simulink model "DemoManipulator"  (R2023a)
settings: Solver=ode23t  StartTime=0.0  StopTime=65  MaxStep=0.01  RelTol=1e-3
undefined symbols (not defined in the file): X, Y, Z
libraries: sm_lib x22, nesl_utility x17
settings Model: Creator=KozlovM  LastModifiedBy=Artem Sannikov

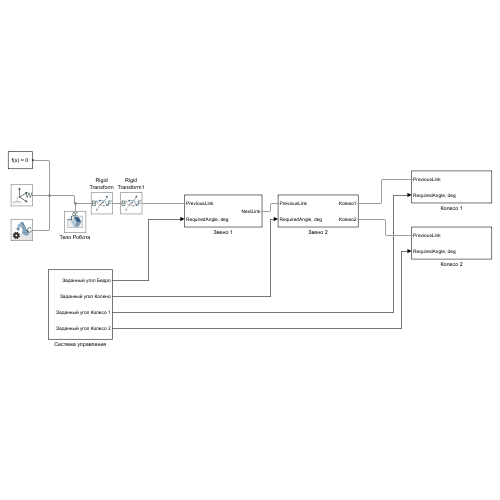
[thumbnail: Simulink's stored preview of the top-level diagram]
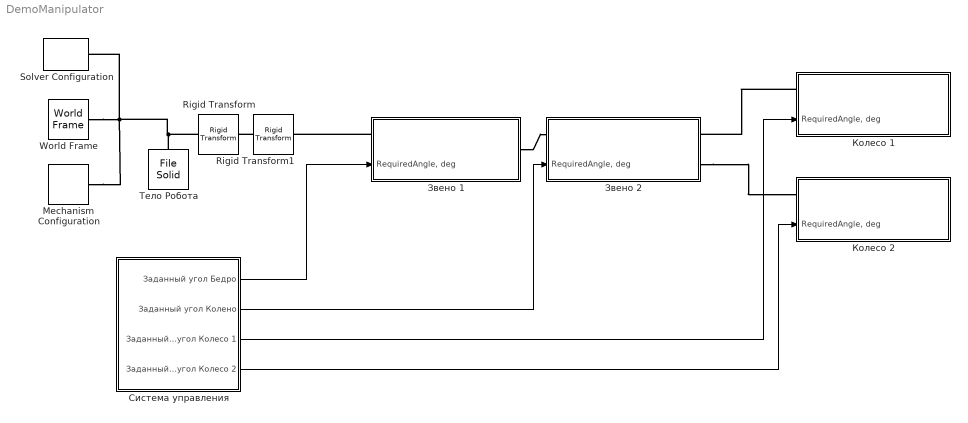
== system DemoManipulator ==
  Mechanism Configuration : sm_lib/Utilities/Mechanism Configuration  UniformGravity=Constant  GravityVector=[0 0 -9.80665]  GravityVectorUnits=m/s^2  LinearizationDelta=0.001  JointModeTransitionNonlinearIterations=2
  Rigid Transform : sm_lib/Frames and Transforms/Rigid Transform  TranslationMethod=StandardAxis  TranslationStandardOffset=117  TranslationStandardOffsetUnits=mm  TranslationStandardAxis=+X  TranslationCartesianOffset=[0 0 0.22]  TranslationCartesianOffsetUnits=m  TranslationROffset=0  TranslationROffsetUnits=m  TranslationZOffset=0  TranslationZOffsetUnits=m  TranslationThetaOffset=0  TranslationThetaOffsetUnits=deg  RotationMethod=None  RotationAngleUnits=deg  RotationStandardAxis=+X  RotationAngle=180  RotationArbitraryAxis=[0 0 1]  FollAlignAxisA=+X  BaseAlignAxisA=+Y  FollAlignAxisB=+Y  BaseAlignAxisB=+Z  RotationSequenceAxes=FollowerAxes  RotationSequence=XYX  RotationSequenceAngles=[0 0 0]  RotationSequenceAnglesUnits=deg  RotationMatrix=[1 0 0; 0 1 0; 0 0 1]  Quaternion=[1 0 0 0]
  Rigid Transform1 : sm_lib/Frames and Transforms/Rigid Transform  TranslationMethod=StandardAxis  TranslationStandardOffset=10  TranslationStandardOffsetUnits=mm  TranslationStandardAxis=-Y  TranslationCartesianOffset=[0 0 0.22]  TranslationCartesianOffsetUnits=m  TranslationROffset=0  TranslationROffsetUnits=m  TranslationZOffset=0  TranslationZOffsetUnits=m  TranslationThetaOffset=0  TranslationThetaOffsetUnits=deg  RotationMethod=None  RotationAngleUnits=deg  RotationStandardAxis=+X  RotationAngle=180  RotationArbitraryAxis=[0 0 1]  FollAlignAxisA=+X  BaseAlignAxisA=+Y  FollAlignAxisB=+Y  BaseAlignAxisB=+Z  RotationSequenceAxes=FollowerAxes  RotationSequence=XYX  RotationSequenceAngles=[0 0 0]  RotationSequenceAnglesUnits=deg  RotationMatrix=[1 0 0; 0 1 0; 0 0 1]  Quaternion=[1 0 0 0]
  Solver Configuration : nesl_utility/Solver Configuration  PhysicalDomain=network_engine_domain  SubClassName=solver  LeftPortType=input  RightPortType=generic  Tones=[]  Harmonics=[]  SimulateNoise=off  Profile=off  UseLocalSampling=off  EnableSwitchedLinearOptims=on  FrequencyDomain=off  UseCCode=off  RelTol=0.001  AbsTol=0.001  MinStep=1e-09  ToWorkspace=off  RevertToSquareIcSolve=off  NumHomotopyIterations=100  PhasorMode=off  PhasorModeNumHarmonics=1  ConsistencySolver=NEWTON_XTOL_AFTER_FTOL  IndexReductionMethod=DerivativeReplacement  DoDC=off  ResidualTolerance=1e-09  ConsistencyTolSource=GLOBAL  ConsistencyAbsTol=0.001  ConsistencyRelTol=0.001  ConsistencyTolFactor=0.001  UseLocalSolver=off  LocalSolverChoice=NE_BACKWARD_EULER_ADVANCER  ResolveIndetEquations=on  FunctionEvalNumThread=1  LocalSolverSampleTime=0.001  DoFixedCost=off  MaxNonlinIter=3  MaxModeIter=2  ComputeImpulses=off  ImpulseIterations=2  LinearAlgebra=auto  LinearAlgebraNumThread=0  EquationFormulation=NE_TIME_EF  DelaysMemoryBudget=1024  AutomaticFiltering=on  FilteringTimeConstant=0.001  PartitionStorageMethod=AS_NEEDED  PartitionMemoryBudget=1024  PartitionMethod=ROBUST
  World Frame : sm_lib/Frames and Transforms/World Frame
  Звено 1 : Subsystem
      settings: PortSchema="{\"entries\":[{\"content\":{\"sides\":[{\"content\":{\"connectorIds\":[\"LConn1\",\"In1\"]},\"type\":\"ConnectorPlacement.EquallySpacedRectSide\",\"uuid\":\"59137c6e-e982-4e9a-8887-9c851b27c4d0\"},{\"content\":{\"connectorIds\":[\"RConn1\"],\"side\":\"RIGHT\"},\"type\":\"ConnectorPlacement.EquallySpacedRectSide\",\"uuid\":\"3006ed02-36e2-47dc-847a-44ef2bf55218\"},{\"content\":{\"side\":\"TOP\"},\"type\":\"ConnectorPlacement.EquallySpacedRectSide\",\"uuid\":\"771aef0a-3ddb-4cfd-8b5b-88211feb2622\"}]},\"type\":\"ConnectorPlacement.EquallySpacedConnector\",\"uuid\":\"e4e6c871-1414-4429-aa1a-adbd621e5483\"}],\"packageUris\":[\"http://schema.mathworks.com/mf0/Connector/R2020b\"],\"version\":\"1.0\"}"
  Звено 2 : Subsystem
      settings: PortSchema="{\"entries\":[{\"content\":{\"sides\":[{\"content\":{\"connectorIds\":[\"LConn1\",\"In1\"]},\"type\":\"ConnectorPlacement.EquallySpacedRectSide\",\"uuid\":\"59137c6e-e982-4e9a-8887-9c851b27c4d0\"},{\"content\":{\"connectorIds\":[\"RConn1\",\"RConn2\"],\"side\":\"RIGHT\"},\"type\":\"ConnectorPlacement.EquallySpacedRectSide\",\"uuid\":\"3006ed02-36e2-47dc-847a-44ef2bf55218\"},{\"content\":{\"side\":\"TOP\"},\"type\":\"ConnectorPlacement.EquallySpacedRectSide\",\"uuid\":\"771aef0a-3ddb-4cfd-8b5b-88211feb2622\"}]},\"type\":\"ConnectorPlacement.EquallySpacedConnector\",\"uuid\":\"e4e6c871-1414-4429-aa1a-adbd621e5483\"}],\"packageUris\":[\"http://schema.mathworks.com/mf0/Connector/R2020b\"],\"version\":\"1.0\"}"
  Колесо 1 : Subsystem
      settings: PortSchema="{\"entries\":[{\"content\":{\"sides\":[{\"content\":{\"connectorIds\":[\"LConn1\",\"In1\"]},\"type\":\"ConnectorPlacement.EquallySpacedRectSide\",\"uuid\":\"59137c6e-e982-4e9a-8887-9c851b27c4d0\"},{\"content\":{\"side\":\"RIGHT\"},\"type\":\"ConnectorPlacement.EquallySpacedRectSide\",\"uuid\":\"3006ed02-36e2-47dc-847a-44ef2bf55218\"},{\"content\":{\"side\":\"TOP\"},\"type\":\"ConnectorPlacement.EquallySpacedRectSide\",\"uuid\":\"771aef0a-3ddb-4cfd-8b5b-88211feb2622\"}]},\"type\":\"ConnectorPlacement.EquallySpacedConnector\",\"uuid\":\"e4e6c871-1414-4429-aa1a-adbd621e5483\"}],\"packageUris\":[\"http://schema.mathworks.com/mf0/Connector/R2020b\"],\"version\":\"1.0\"}"
  Колесо 2 : Subsystem
      settings: PortSchema="{\"entries\":[{\"content\":{\"sides\":[{\"content\":{\"connectorIds\":[\"LConn1\",\"In1\"]},\"type\":\"ConnectorPlacement.EquallySpacedRectSide\",\"uuid\":\"59137c6e-e982-4e9a-8887-9c851b27c4d0\"},{\"content\":{\"side\":\"RIGHT\"},\"type\":\"ConnectorPlacement.EquallySpacedRectSide\",\"uuid\":\"3006ed02-36e2-47dc-847a-44ef2bf55218\"},{\"content\":{\"side\":\"TOP\"},\"type\":\"ConnectorPlacement.EquallySpacedRectSide\",\"uuid\":\"771aef0a-3ddb-4cfd-8b5b-88211feb2622\"}]},\"type\":\"ConnectorPlacement.EquallySpacedConnector\",\"uuid\":\"e4e6c871-1414-4429-aa1a-adbd621e5483\"}],\"packageUris\":[\"http://schema.mathworks.com/mf0/Connector/R2020b\"],\"version\":\"1.0\"}"
  Система управления : Subsystem
  Тело Робота : sm_lib/Body Elements/File Solid  ExtGeomFileName=C:\Users\Artem Sannikov\Desktop\Robo-Forester\Simulink_часть\3D_Models\Body.stp  UnitType=FromFile  ExtGeomFileUnits=ft  StepReaderType=HEX  ExportConvexHullGeometry=off  InertiaType=Custom  Mass=1000  MassUnits=kg  CenterOfMass=[0 0 0]  CenterOfMassUnits=m  MomentsOfInertia=[1 1 1]  MomentsOfInertiaUnits=kg*m^2  ProductsOfInertia=[0 0 0]  ProductsOfInertiaUnits=kg*m^2  BasedOnType=Mass  Density=1000  DensityUnits=kg/m^3  DoExposeReferenceFrame=on  SerializedFrames=<Frames/>  GraphicType=FromGeometry  MarkerShape=Sphere  MarkerSize=10  GraphicVisPropType=SimpleVisualProperties  GraphicDiffuseColor=[0.5 0.5 0.5]  GraphicSpecularColor=[0.5 0.5 0.5 1.0]  GraphicAmbientColor=[0.15 0.15 0.15 1.0]  GraphicEmissiveColor=[0.0 0.0 0.0 1.0]  GraphicShininess=75  GraphicOpacity=1.0
  wires:
  Система управления/1(Заданный угол Бедро) -> Звено 1/1("RequiredAngle, deg")
  Система управления/2(Заданный угол Колено) -> Звено 2/1("RequiredAngle, deg")
  Система управления/3(Заданный угол Колесо 1) -> Колесо 1/1("RequiredAngle, deg")
  Система управления/4(Заданный угол Колесо 2) -> Колесо 2/1("RequiredAngle, deg")
  connections:
  Звено 1/LConn1 -- Rigid Transform1/RConn1
  Звено 1/RConn1 -- Звено 2/LConn1
  Колесо 1/LConn1 -- Звено 2/RConn1
  Rigid Transform/LConn1 -- Mechanism Configuration/RConn1 -- World Frame/RConn1 -- Solver Configuration/RConn1 -- Тело Робота/RConn1
  Rigid Transform1/LConn1 -- Rigid Transform/RConn1
  Звено 2/RConn2 -- Колесо 2/LConn1

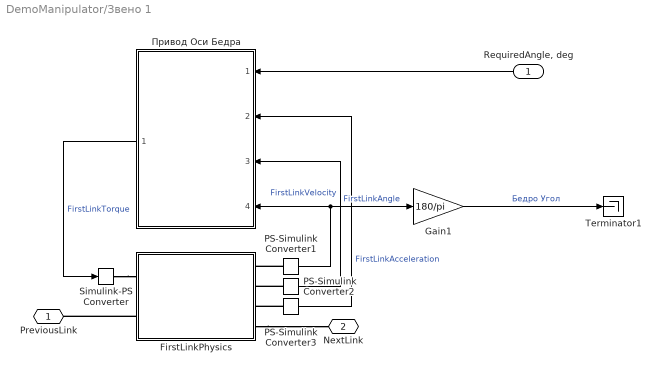
== system DemoManipulator/Звено 1 ==
  "RequiredAngle, deg" : Inport
  FirstLinkPhysics : Subsystem
  Gain1 : Gain  Gain=180/pi
  PS-Simulink Converter1 : nesl_utility/PS-Simulink Converter  PhysicalDomain=network_engine_domain  SubClassName=ps_output  LeftPortType=input  RightPortType=output  PseudoPeriodic=off  Frequencies=[]  VectorFormat=inherit  Unit=inherit  AffineConversion=off
  PS-Simulink Converter2 : nesl_utility/PS-Simulink Converter  PhysicalDomain=network_engine_domain  SubClassName=ps_output  LeftPortType=input  RightPortType=output  PseudoPeriodic=off  Frequencies=[]  VectorFormat=inherit  Unit=inherit  AffineConversion=off
  PS-Simulink Converter3 : nesl_utility/PS-Simulink Converter  PhysicalDomain=network_engine_domain  SubClassName=ps_output  LeftPortType=input  RightPortType=output  PseudoPeriodic=off  Frequencies=[]  VectorFormat=inherit  Unit=inherit  AffineConversion=off
  Simulink-PS Converter : nesl_utility/Simulink-PS Converter  PhysicalDomain=network_engine_domain  SubClassName=ps_input  LeftPortType=input  RightPortType=output  PseudoPeriodic=off  Frequencies=[]  NoiseDistribution=none  NoiseParameters=[]  Unit=1  AffineConversion=off  FilteringAndDerivatives=provide  SimscapeFilterOrder=1  InputFilterTimeConstant=0.001  UdotUserProvided=0
  Terminator1 : Terminator
  Привод Оси Бедра : Subsystem  TreatAsAtomicUnit=on  ReferencedSubsystem=Actuator  K=10  Kv=10  K1=0.05  K2=10  K3=300
  PreviousLink : PMIOPort  Side=Left
  NextLink : PMIOPort  Port=2  Side=Right
  wires:
  Привод Оси Бедра/1 -> Simulink-PS Converter/1  "FirstLinkTorque"
  PS-Simulink Converter1/1 -> Gain1/1, Привод Оси Бедра/4  "FirstLinkAngle"
  PS-Simulink Converter2/1 -> Привод Оси Бедра/3  "FirstLinkVelocity"
  PS-Simulink Converter3/1 -> Привод Оси Бедра/2  "FirstLinkAcceleration"
  "RequiredAngle, deg"/1 -> Привод Оси Бедра/1
  Gain1/1 -> Terminator1/1  "Бедро Угол"
  connections:
  PS-Simulink Converter1/LConn1 -- FirstLinkPhysics/RConn1
  PS-Simulink Converter3/LConn1 -- FirstLinkPhysics/RConn3
  Simulink-PS Converter/RConn1 -- FirstLinkPhysics/LConn1
  PS-Simulink Converter2/LConn1 -- FirstLinkPhysics/RConn2
  FirstLinkPhysics/LConn2 -- PreviousLink/RConn1
  FirstLinkPhysics/RConn4 -- NextLink/RConn1

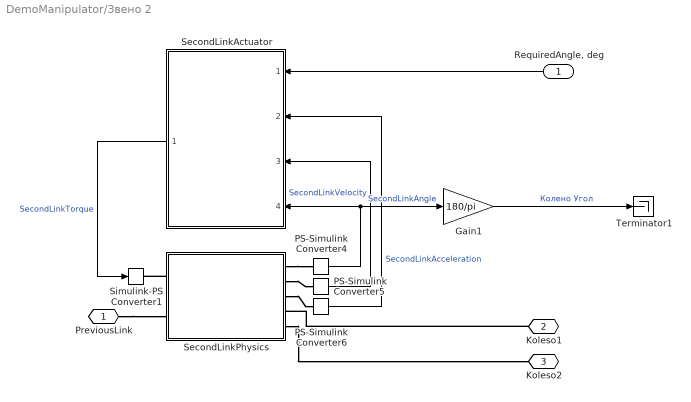
== system DemoManipulator/Звено 2 ==
  "RequiredAngle, deg" : Inport
  Gain1 : Gain  Gain=180/pi
  PS-Simulink Converter4 : nesl_utility/PS-Simulink Converter  PhysicalDomain=network_engine_domain  SubClassName=ps_output  LeftPortType=input  RightPortType=output  PseudoPeriodic=off  Frequencies=[]  VectorFormat=inherit  Unit=inherit  AffineConversion=off
  PS-Simulink Converter5 : nesl_utility/PS-Simulink Converter  PhysicalDomain=network_engine_domain  SubClassName=ps_output  LeftPortType=input  RightPortType=output  PseudoPeriodic=off  Frequencies=[]  VectorFormat=inherit  Unit=inherit  AffineConversion=off
  PS-Simulink Converter6 : nesl_utility/PS-Simulink Converter  PhysicalDomain=network_engine_domain  SubClassName=ps_output  LeftPortType=input  RightPortType=output  PseudoPeriodic=off  Frequencies=[]  VectorFormat=inherit  Unit=inherit  AffineConversion=off
  SecondLinkActuator : Subsystem  TreatAsAtomicUnit=on  ReferencedSubsystem=Actuator  K=10  Kv=15  K1=0.05  K2=50  K3=100
  SecondLinkPhysics : Subsystem
  Simulink-PS Converter1 : nesl_utility/Simulink-PS Converter  PhysicalDomain=network_engine_domain  SubClassName=ps_input  LeftPortType=input  RightPortType=output  PseudoPeriodic=off  Frequencies=[]  NoiseDistribution=none  NoiseParameters=[]  Unit=1  AffineConversion=off  FilteringAndDerivatives=provide  SimscapeFilterOrder=1  InputFilterTimeConstant=0.001  UdotUserProvided=0
  Terminator1 : Terminator
  PreviousLink : PMIOPort  Side=Left
  Koleso1 : PMIOPort  Port=2  Side=Right
  Koleso2 : PMIOPort  Port=3  Side=Right
  wires:
  SecondLinkActuator/1 -> Simulink-PS Converter1/1  "SecondLinkTorque"
  PS-Simulink Converter5/1 -> SecondLinkActuator/3  "SecondLinkVelocity"
  PS-Simulink Converter6/1 -> SecondLinkActuator/2  "SecondLinkAcceleration"
  "RequiredAngle, deg"/1 -> SecondLinkActuator/1
  Gain1/1 -> Terminator1/1  "Колено Угол"
  PS-Simulink Converter4/1 -> SecondLinkActuator/4, Gain1/1  "SecondLinkAngle"
  connections:
  SecondLinkPhysics/RConn1 -- PS-Simulink Converter4/LConn1
  SecondLinkPhysics/RConn2 -- PS-Simulink Converter5/LConn1
  SecondLinkPhysics/LConn1 -- Simulink-PS Converter1/RConn1
  SecondLinkPhysics/RConn3 -- PS-Simulink Converter6/LConn1
  Koleso1/RConn1 -- SecondLinkPhysics/RConn4
  PreviousLink/RConn1 -- SecondLinkPhysics/LConn2
  SecondLinkPhysics/RConn5 -- Koleso2/RConn1

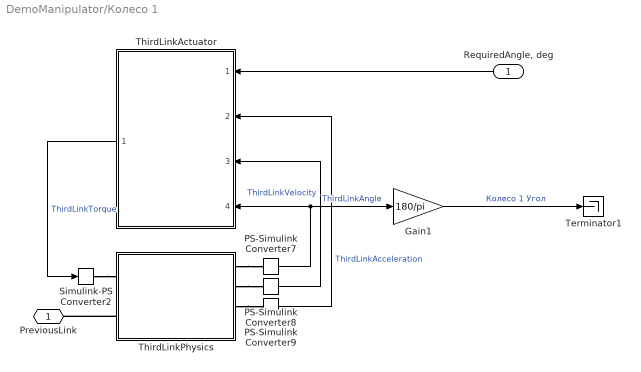
== system DemoManipulator/Колесо 1 ==
  "RequiredAngle, deg" : Inport
  Gain1 : Gain  Gain=180/pi
  PS-Simulink Converter7 : nesl_utility/PS-Simulink Converter  PhysicalDomain=network_engine_domain  SubClassName=ps_output  LeftPortType=input  RightPortType=output  PseudoPeriodic=off  Frequencies=[]  VectorFormat=inherit  Unit=inherit  AffineConversion=off
  PS-Simulink Converter8 : nesl_utility/PS-Simulink Converter  PhysicalDomain=network_engine_domain  SubClassName=ps_output  LeftPortType=input  RightPortType=output  PseudoPeriodic=off  Frequencies=[]  VectorFormat=inherit  Unit=inherit  AffineConversion=off
  PS-Simulink Converter9 : nesl_utility/PS-Simulink Converter  PhysicalDomain=network_engine_domain  SubClassName=ps_output  LeftPortType=input  RightPortType=output  PseudoPeriodic=off  Frequencies=[]  VectorFormat=inherit  Unit=inherit  AffineConversion=off
  Simulink-PS Converter2 : nesl_utility/Simulink-PS Converter  PhysicalDomain=network_engine_domain  SubClassName=ps_input  LeftPortType=input  RightPortType=output  PseudoPeriodic=off  Frequencies=[]  NoiseDistribution=none  NoiseParameters=[]  Unit=1  AffineConversion=off  FilteringAndDerivatives=provide  SimscapeFilterOrder=1  InputFilterTimeConstant=0.001  UdotUserProvided=0
  Terminator1 : Terminator
  ThirdLinkActuator : Subsystem  TreatAsAtomicUnit=on  ReferencedSubsystem=Actuator  K=10  Kv=10  K1=0.05  K2=10  K3=1000
  ThirdLinkPhysics : Subsystem
  PreviousLink : PMIOPort  Side=Left
  wires:
  ThirdLinkActuator/1 -> Simulink-PS Converter2/1  "ThirdLinkTorque"
  PS-Simulink Converter7/1 -> Gain1/1, ThirdLinkActuator/4  "ThirdLinkAngle"
  PS-Simulink Converter9/1 -> ThirdLinkActuator/2  "ThirdLinkAcceleration"
  PS-Simulink Converter8/1 -> ThirdLinkActuator/3  "ThirdLinkVelocity"
  Gain1/1 -> Terminator1/1  "Колесо 1 Угол"
  "RequiredAngle, deg"/1 -> ThirdLinkActuator/1
  connections:
  ThirdLinkPhysics/RConn3 -- PS-Simulink Converter9/LConn1
  Simulink-PS Converter2/RConn1 -- ThirdLinkPhysics/LConn1
  ThirdLinkPhysics/RConn2 -- PS-Simulink Converter8/LConn1
  ThirdLinkPhysics/RConn1 -- PS-Simulink Converter7/LConn1
  ThirdLinkPhysics/LConn2 -- PreviousLink/RConn1

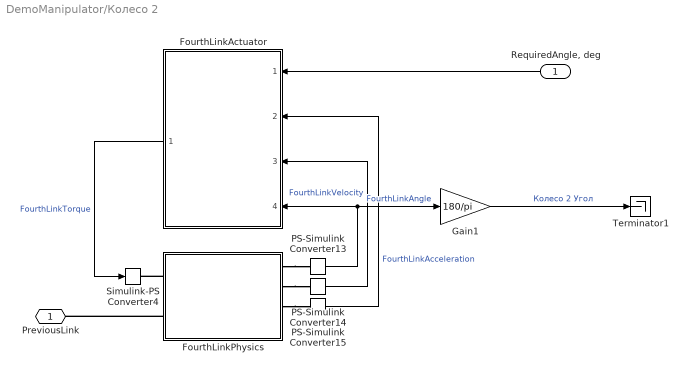
== system DemoManipulator/Колесо 2 ==
  "RequiredAngle, deg" : Inport
  FourthLinkActuator : Subsystem  TreatAsAtomicUnit=on  ReferencedSubsystem=Actuator  K=10  Kv=10  K1=0.05  K2=10  K3=100
  FourthLinkPhysics : Subsystem
  Gain1 : Gain  Gain=180/pi
  PS-Simulink Converter13 : nesl_utility/PS-Simulink Converter  PhysicalDomain=network_engine_domain  SubClassName=ps_output  LeftPortType=input  RightPortType=output  PseudoPeriodic=off  Frequencies=[]  VectorFormat=inherit  Unit=inherit  AffineConversion=off
  PS-Simulink Converter14 : nesl_utility/PS-Simulink Converter  PhysicalDomain=network_engine_domain  SubClassName=ps_output  LeftPortType=input  RightPortType=output  PseudoPeriodic=off  Frequencies=[]  VectorFormat=inherit  Unit=inherit  AffineConversion=off
  PS-Simulink Converter15 : nesl_utility/PS-Simulink Converter  PhysicalDomain=network_engine_domain  SubClassName=ps_output  LeftPortType=input  RightPortType=output  PseudoPeriodic=off  Frequencies=[]  VectorFormat=inherit  Unit=inherit  AffineConversion=off
  Simulink-PS Converter4 : nesl_utility/Simulink-PS Converter  PhysicalDomain=network_engine_domain  SubClassName=ps_input  LeftPortType=input  RightPortType=output  PseudoPeriodic=off  Frequencies=[]  NoiseDistribution=none  NoiseParameters=[]  Unit=1  AffineConversion=off  FilteringAndDerivatives=provide  SimscapeFilterOrder=1  InputFilterTimeConstant=0.001  UdotUserProvided=0
  Terminator1 : Terminator
  PreviousLink : PMIOPort  Side=Left
  wires:
  FourthLinkActuator/1 -> Simulink-PS Converter4/1  "FourthLinkTorque"
  PS-Simulink Converter14/1 -> FourthLinkActuator/3  "FourthLinkVelocity"
  PS-Simulink Converter15/1 -> FourthLinkActuator/2  "FourthLinkAcceleration"
  Gain1/1 -> Terminator1/1  "Колесо 2 Угол"
  PS-Simulink Converter13/1 -> FourthLinkActuator/4, Gain1/1  "FourthLinkAngle"
  "RequiredAngle, deg"/1 -> FourthLinkActuator/1
  connections:
  FourthLinkPhysics/LConn1 -- Simulink-PS Converter4/RConn1
  FourthLinkPhysics/RConn2 -- PS-Simulink Converter14/LConn1
  FourthLinkPhysics/RConn1 -- PS-Simulink Converter13/LConn1
  FourthLinkPhysics/RConn3 -- PS-Simulink Converter15/LConn1
  FourthLinkPhysics/LConn2 -- PreviousLink/RConn1

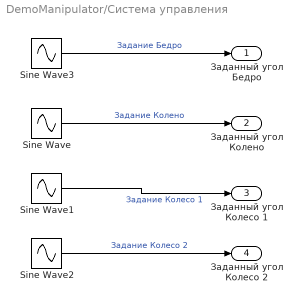
== system DemoManipulator/Система управления ==
  Sine Wave : Sin  Amplitude=180  Bias=60  Frequency=0.5  SampleTime=0
  Sine Wave1 : Sin  Amplitude=30  Bias=40  SampleTime=0
  Sine Wave2 : Sin  Amplitude=30  Bias=40  SampleTime=0
  Sine Wave3 : Sin  Amplitude=40  Bias=60  Frequency=0.5  SampleTime=0
  Заданный угол Бедро : Outport
  Заданный угол Колено : Outport  Port=2
  Заданный угол Колесо 1 : Outport  Port=3
  Заданный угол Колесо 2 : Outport  Port=4
  wires:
  Sine Wave/1 -> Заданный угол Колено/1  "Задание Колено"
  Sine Wave3/1 -> Заданный угол Бедро/1  "Задание Бедро"
  Sine Wave2/1 -> Заданный угол Колесо 2/1  "Задание Колесо 2"
  Sine Wave1/1 -> Заданный угол Колесо 1/1  "Задание Колесо 1"

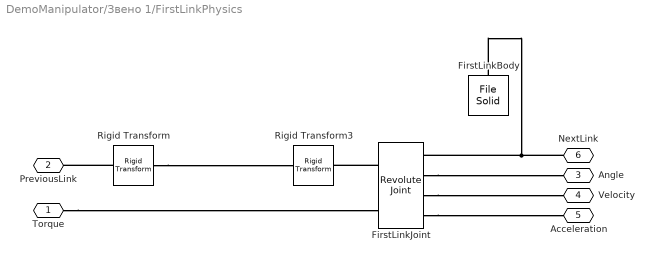
== system DemoManipulator/Звено 1/FirstLinkPhysics ==
  FirstLinkBody : sm_lib/Body Elements/File Solid  ExtGeomFileName=C:\Users\Artem Sannikov\Desktop\Robo-Forester\Simulink_часть\3D_Models\Leg.stp  UnitType=FromFile  ExtGeomFileUnits=m  StepReaderType=HEX  ExportConvexHullGeometry=off  InertiaType=Custom  Mass=5.3  MassUnits=kg  CenterOfMass=[0 0 -90]  CenterOfMassUnits=mm  MomentsOfInertia=[15.3 20.5 5.7]  MomentsOfInertiaUnits=kg*m^2  ProductsOfInertia=[0 0 0]  ProductsOfInertiaUnits=kg*m^2  BasedOnType=DensityFromFile  Density=1000  DensityUnits=kg/m^3  DoExposeReferenceFrame=on  SerializedFrames=<Frames><Frame><Id>Frame1</Id><Value><Name>Bedro</Name><Origin><Source>GeometricFeature</Source><FeatureName>cylindrical surface 7</FeatureName></Origin><PrimaryAxis><DefinedDirection>+Z</DefinedDirection><Source>GeometricFeature</Source><SourceDirection>+Z</SourceDirection><FeatureName>cylindrical surface 7</FeatureName></PrimaryAxis><SecondaryAxis><DefinedDirection>+X</DefinedDirection><Source>GeometricFeature</Source><SourceDirection>+X</SourceDirection><FeatureName></FeatureName></SecondaryAxis></Value></Frame></Frames>  GraphicType=FromGeometry  MarkerShape=Sphere  MarkerSize=10  GraphicVisPropType=FromFileVisualProperties  GraphicDiffuseColor=[0.5 0.5 0.5]  GraphicSpecularColor=[0.5 0.5 0.5 1.0]  GraphicAmbientColor=[0.15 0.15 0.15 1.0]  GraphicEmissiveColor=[0.0 0.0 0.0 1.0]  GraphicShininess=75  GraphicOpacity=1.0
  FirstLinkJoint : sm_lib/Joints/Revolute Joint  JointMode=Normal  SenseConstraintForce=off  SenseConstraintForceX=off  SenseConstraintForceY=off  SenseConstraintForceZ=off  SenseConstraintTorque=off  SenseConstraintTorqueX=off  SenseConstraintTorqueY=off  SenseConstraintTorqueZ=off  SenseTotalForce=off  SenseTotalForceX=off  SenseTotalForceY=off  SenseTotalForceZ=off  SenseTotalTorque=off  SenseTotalTorqueX=off  SenseTotalTorqueY=off  SenseTotalTorqueZ=off  CompositeWrenchDir=FollowerOnBase  CompositeWrenchFrame=BaseFrame  EquilibriumPosition=0  EquilibriumPositionUnits=deg  SpringStiffness=0  SpringStiffnessUnits=N*m/deg  DampingCoefficient=0.1  DampingCoefficientUnits=N*m/(deg/s)  TorqueActuationMode=InputTorque  MotionActuationMode=ComputedMotion  SensePosition=on  SenseVelocity=on  SenseAcceleration=on  SenseTorqueForce=off  SenseLowerLimitTorqueForce=off  SenseUpperLimitTorqueForce=off  LowerLimitSpecify=on  LowerLimitBound=-170  LowerLimitBoundUnits=deg  LowerLimitStiffness=1e4  LowerLimitStiffnessUnits=N*m/deg  LowerLimitDamping=1000  LowerLimitDampingUnits=N*m/(deg/s)  LowerLimitTransitionRegionWidth=0.1  LowerLimitTransitionRegionWidthUnits=deg  UpperLimitSpecify=on  UpperLimitBound=170  UpperLimitBoundUnits=deg  UpperLimitStiffness=1e4  UpperLimitStiffnessUnits=N*m/deg  UpperLimitDamping=1000  UpperLimitDampingUnits=N*m/(deg/s)  UpperLimitTransitionRegionWidth=0.1  UpperLimitTransitionRegionWidthUnits=deg  PositionTargetSpecify=on  PositionTargetPriority=High  PositionTargetValue=0  PositionTargetValueUnits=deg  VelocityTargetSpecify=off  VelocityTargetPriority=High  VelocityTargetValue=0  VelocityTargetValueUnits=deg/s
  Rigid Transform : sm_lib/Frames and Transforms/Rigid Transform  TranslationMethod=None  TranslationStandardOffset=0  TranslationStandardOffsetUnits=m  TranslationStandardAxis=+Z  TranslationCartesianOffset=[0 0 0.22]  TranslationCartesianOffsetUnits=m  TranslationROffset=0  TranslationROffsetUnits=m  TranslationZOffset=0  TranslationZOffsetUnits=m  TranslationThetaOffset=0  TranslationThetaOffsetUnits=deg  RotationMethod=StandardAxis  RotationAngleUnits=deg  RotationStandardAxis=-Z  RotationAngle=45  RotationArbitraryAxis=[0 0 1]  FollAlignAxisA=+X  BaseAlignAxisA=+Y  FollAlignAxisB=+Y  BaseAlignAxisB=+Z  RotationSequenceAxes=FollowerAxes  RotationSequence=XYX  RotationSequenceAngles=[0 0 0]  RotationSequenceAnglesUnits=deg  RotationMatrix=[1 0 0; 0 1 0; 0 0 1]  Quaternion=[1 0 0 0]
  Rigid Transform3 : sm_lib/Frames and Transforms/Rigid Transform  TranslationMethod=StandardAxis  TranslationStandardOffset=10  TranslationStandardOffsetUnits=mm  TranslationStandardAxis=+Z  TranslationCartesianOffset=[0 0 0.22]  TranslationCartesianOffsetUnits=m  TranslationROffset=0  TranslationROffsetUnits=m  TranslationZOffset=0  TranslationZOffsetUnits=m  TranslationThetaOffset=0  TranslationThetaOffsetUnits=deg  RotationMethod=None  RotationAngleUnits=deg  RotationStandardAxis=+X  RotationAngle=180  RotationArbitraryAxis=[0 0 1]  FollAlignAxisA=+X  BaseAlignAxisA=+Y  FollAlignAxisB=+Y  BaseAlignAxisB=+Z  RotationSequenceAxes=FollowerAxes  RotationSequence=XYX  RotationSequenceAngles=[0 0 0]  RotationSequenceAnglesUnits=deg  RotationMatrix=[1 0 0; 0 1 0; 0 0 1]  Quaternion=[1 0 0 0]
  Torque : PMIOPort  Side=Left
  PreviousLink : PMIOPort  Port=2  Side=Left
  Angle : PMIOPort  Port=3  Side=Right
  Velocity : PMIOPort  Port=4  Side=Right
  Acceleration : PMIOPort  Port=5  Side=Right
  NextLink : PMIOPort  Port=6  Side=Right
  connections:
  FirstLinkJoint/RConn2 -- Angle/RConn1
  FirstLinkJoint/RConn4 -- Acceleration/RConn1
  FirstLinkJoint/RConn3 -- Velocity/RConn1
  NextLink/RConn1 -- FirstLinkBody/LConn1 -- FirstLinkJoint/RConn1
  FirstLinkJoint/LConn1 -- Rigid Transform3/RConn1
  Torque/RConn1 -- FirstLinkJoint/LConn2
  Rigid Transform/LConn1 -- PreviousLink/RConn1
  Rigid Transform/RConn1 -- Rigid Transform3/LConn1

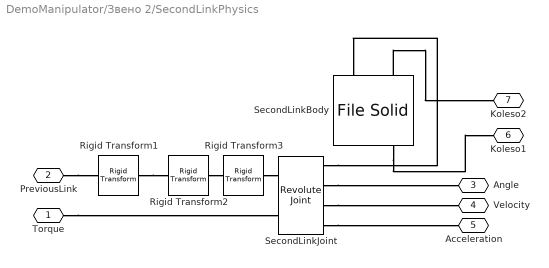
== system DemoManipulator/Звено 2/SecondLinkPhysics ==
  Rigid Transform1 : sm_lib/Frames and Transforms/Rigid Transform  TranslationMethod=StandardAxis  TranslationStandardOffset=110  TranslationStandardOffsetUnits=mm  TranslationStandardAxis=-Y  TranslationCartesianOffset=[0 0 0.22]  TranslationCartesianOffsetUnits=m  TranslationROffset=0  TranslationROffsetUnits=m  TranslationZOffset=0  TranslationZOffsetUnits=m  TranslationThetaOffset=0  TranslationThetaOffsetUnits=deg  RotationMethod=None  RotationAngleUnits=deg  RotationStandardAxis=+X  RotationAngle=180  RotationArbitraryAxis=[0 0 1]  FollAlignAxisA=+X  BaseAlignAxisA=+Y  FollAlignAxisB=+Y  BaseAlignAxisB=+Z  RotationSequenceAxes=FollowerAxes  RotationSequence=XYX  RotationSequenceAngles=[0 0 0]  RotationSequenceAnglesUnits=deg  RotationMatrix=[1 0 0; 0 1 0; 0 0 1]  Quaternion=[1 0 0 0]
  Rigid Transform2 : sm_lib/Frames and Transforms/Rigid Transform  TranslationMethod=StandardAxis  TranslationStandardOffset=221  TranslationStandardOffsetUnits=mm  TranslationStandardAxis=-X  TranslationCartesianOffset=[0 0 0.22]  TranslationCartesianOffsetUnits=m  TranslationROffset=0  TranslationROffsetUnits=m  TranslationZOffset=0  TranslationZOffsetUnits=m  TranslationThetaOffset=0  TranslationThetaOffsetUnits=deg  RotationMethod=None  RotationAngleUnits=deg  RotationStandardAxis=+X  RotationAngle=180  RotationArbitraryAxis=[0 0 1]  FollAlignAxisA=+X  BaseAlignAxisA=+Y  FollAlignAxisB=+Y  BaseAlignAxisB=+Z  RotationSequenceAxes=FollowerAxes  RotationSequence=XYX  RotationSequenceAngles=[0 0 0]  RotationSequenceAnglesUnits=deg  RotationMatrix=[1 0 0; 0 1 0; 0 0 1]  Quaternion=[1 0 0 0]
  Rigid Transform3 : sm_lib/Frames and Transforms/Rigid Transform  TranslationMethod=StandardAxis  TranslationStandardOffset=75  TranslationStandardOffsetUnits=mm  TranslationStandardAxis=-Z  TranslationCartesianOffset=[0 0 0.22]  TranslationCartesianOffsetUnits=m  TranslationROffset=0  TranslationROffsetUnits=m  TranslationZOffset=0  TranslationZOffsetUnits=m  TranslationThetaOffset=0  TranslationThetaOffsetUnits=deg  RotationMethod=None  RotationAngleUnits=deg  RotationStandardAxis=+X  RotationAngle=180  RotationArbitraryAxis=[0 0 1]  FollAlignAxisA=+X  BaseAlignAxisA=+Y  FollAlignAxisB=+Y  BaseAlignAxisB=+Z  RotationSequenceAxes=FollowerAxes  RotationSequence=XYX  RotationSequenceAngles=[0 0 0]  RotationSequenceAnglesUnits=deg  RotationMatrix=[1 0 0; 0 1 0; 0 0 1]  Quaternion=[1 0 0 0]
  SecondLinkBody : sm_lib/Body Elements/File Solid  ExtGeomFileName=C:\Users\Artem Sannikov\Desktop\Robo-Forester\Simulink_часть\3D_Models\knee.stp  UnitType=FromFile  ExtGeomFileUnits=m  StepReaderType=HEX  ExportConvexHullGeometry=off  InertiaType=Custom  Mass=2  MassUnits=kg  CenterOfMass=[-100 0 0]  CenterOfMassUnits=mm  MomentsOfInertia=[13.4 18.7 6.4]  MomentsOfInertiaUnits=kg*m^2  ProductsOfInertia=[0 0 0]  ProductsOfInertiaUnits=kg*m^2  BasedOnType=DensityFromFile  Density=1000  DensityUnits=kg/m^3  DoExposeReferenceFrame=on  SerializedFrames=<Frames><Frame><Id>Frame1</Id><Value><Name>Koleno</Name><Origin><Source>GeometricFeature</Source><FeatureName>planar surface 1</FeatureName></Origin><PrimaryAxis><DefinedDirection>+Z</DefinedDirection><Source>GeometricFeature</Source><SourceDirection>+Z</SourceDirection><FeatureName>planar surface 1</FeatureName></PrimaryAxis><SecondaryAxis><DefinedDirection>+X</DefinedDirection><Source>ReferenceFrame</Source><SourceDirection>+X</SourceDirection><FeatureName></FeatureName></SecondaryAxis></Value></Frame><Frame><Id>Frame2</Id><Value><Name>Koleso2</Name><Origin><Source>GeometricFeature</Source><FeatureName>planar surface 2</FeatureName></Origin><PrimaryAxis><DefinedDirection>+Z</DefinedDirection><Source>ReferenceFrame</Source><SourceDirection>+Z</SourceDirection><FeatureName></FeatureName></PrimaryAxis><SecondaryAxis><DefinedDirection>+X</DefinedDirection><Source>ReferenceFrame</Source><SourceDirection>+X</SourceDirection><FeatureName></FeatureName></SecondaryAxis></Value></Frame><Frame><Id>Frame3</Id><Value><Name>Koleso1</Name><Origin><Source>GeometricFeature</Source><FeatureName>planar surface 7</FeatureName></Origin><PrimaryAxis><DefinedDirection>+Z</DefinedDirection><Source>ReferenceFrame</Source><SourceDirection>+Z</SourceDirection><FeatureName></FeatureName></PrimaryAxis><SecondaryAxis><DefinedDirection>+X</DefinedDirection><Source>ReferenceFrame</Source><SourceDirection>+X</SourceDirection><FeatureName></FeatureName></SecondaryAxis></Value></Frame></Frames>  GraphicType=FromGeometry  MarkerShape=Sphere  MarkerSize=10  GraphicVisPropType=SimpleVisualProperties  GraphicDiffuseColor=[0.5 0.5 0.5]  GraphicSpecularColor=[0.5 0.5 0.5 1.0]  GraphicAmbientColor=[0.15 0.15 0.15 1.0]  GraphicEmissiveColor=[0.0 0.0 0.0 1.0]  GraphicShininess=75  GraphicOpacity=1.0
  SecondLinkJoint : sm_lib/Joints/Revolute Joint  JointMode=Normal  SenseConstraintForce=off  SenseConstraintForceX=off  SenseConstraintForceY=off  SenseConstraintForceZ=off  SenseConstraintTorque=off  SenseConstraintTorqueX=off  SenseConstraintTorqueY=off  SenseConstraintTorqueZ=off  SenseTotalForce=off  SenseTotalForceX=off  SenseTotalForceY=off  SenseTotalForceZ=off  SenseTotalTorque=off  SenseTotalTorqueX=off  SenseTotalTorqueY=off  SenseTotalTorqueZ=off  CompositeWrenchDir=FollowerOnBase  CompositeWrenchFrame=BaseFrame  EquilibriumPosition=0  EquilibriumPositionUnits=deg  SpringStiffness=0  SpringStiffnessUnits=N*m/deg  DampingCoefficient=0.1  DampingCoefficientUnits=N*m/(deg/s)  TorqueActuationMode=InputTorque  MotionActuationMode=ComputedMotion  SensePosition=on  SenseVelocity=on  SenseAcceleration=on  SenseTorqueForce=off  SenseLowerLimitTorqueForce=off  SenseUpperLimitTorqueForce=off  LowerLimitSpecify=on  LowerLimitBound=-170  LowerLimitBoundUnits=deg  LowerLimitStiffness=1e4  LowerLimitStiffnessUnits=N*m/deg  LowerLimitDamping=1000  LowerLimitDampingUnits=N*m/(deg/s)  LowerLimitTransitionRegionWidth=0.1  LowerLimitTransitionRegionWidthUnits=deg  UpperLimitSpecify=on  UpperLimitBound=50  UpperLimitBoundUnits=deg  UpperLimitStiffness=1e4  UpperLimitStiffnessUnits=N*m/deg  UpperLimitDamping=10  UpperLimitDampingUnits=N*m/(deg/s)  UpperLimitTransitionRegionWidth=0.1  UpperLimitTransitionRegionWidthUnits=deg  PositionTargetSpecify=on  PositionTargetPriority=High  PositionTargetValue=-90  PositionTargetValueUnits=deg  VelocityTargetSpecify=off  VelocityTargetPriority=High  VelocityTargetValue=0  VelocityTargetValueUnits=deg/s
  Torque : PMIOPort  Side=Left
  PreviousLink : PMIOPort  Port=2  Side=Left
  Angle : PMIOPort  Port=3  Side=Right
  Velocity : PMIOPort  Port=4  Side=Right
  Acceleration : PMIOPort  Port=5  Side=Right
  Koleso1 : PMIOPort  Port=6  Side=Right
  Koleso2 : PMIOPort  Port=7  Side=Right
  connections:
  SecondLinkJoint/RConn2 -- Angle/RConn1
  SecondLinkJoint/RConn4 -- Acceleration/RConn1
  SecondLinkJoint/RConn3 -- Velocity/RConn1
  SecondLinkJoint/RConn1 -- SecondLinkBody/LConn1
  Rigid Transform2/RConn1 -- Rigid Transform3/LConn1
  Torque/RConn1 -- SecondLinkJoint/LConn2
  PreviousLink/RConn1 -- Rigid Transform1/LConn1
  Rigid Transform1/RConn1 -- Rigid Transform2/LConn1
  Rigid Transform3/RConn1 -- SecondLinkJoint/LConn1
  SecondLinkBody/LConn2 -- Koleso2/RConn1
  SecondLinkBody/RConn2 -- Koleso1/RConn1

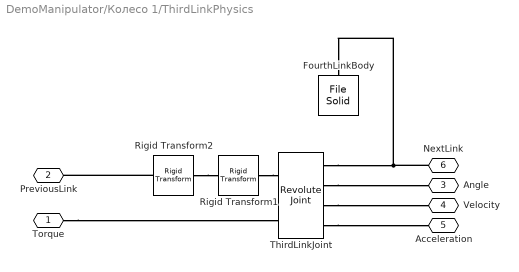
== system DemoManipulator/Колесо 1/ThirdLinkPhysics ==
  FourthLinkBody : sm_lib/Body Elements/File Solid  ExtGeomFileName=C:\Users\Artem Sannikov\Desktop\Robo-Forester\Simulink_часть\3D_Models\Wheel.stp  UnitType=FromFile  ExtGeomFileUnits=m  StepReaderType=HEX  ExportConvexHullGeometry=off  InertiaType=Custom  Mass=1  MassUnits=kg  CenterOfMass=[0 0 -50]  CenterOfMassUnits=m  MomentsOfInertia=[5.7 15.3 4.1]  MomentsOfInertiaUnits=kg*m^2  ProductsOfInertia=[0 0 0]  ProductsOfInertiaUnits=kg*m^2  BasedOnType=DensityFromFile  Density=1000  DensityUnits=kg/m^3  DoExposeReferenceFrame=on  SerializedFrames=<Frames><Frame><Id>Frame1</Id><Value><Name>F1</Name><Origin><Source>GeometricFeature</Source><FeatureName>circular curve 3499</FeatureName></Origin><PrimaryAxis><DefinedDirection>+Z</DefinedDirection><Source>GeometricFeature</Source><SourceDirection>+Z</SourceDirection><FeatureName>segment 2464</FeatureName></PrimaryAxis><SecondaryAxis><DefinedDirection>+X</DefinedDirection><Source>ReferenceFrame</Source><SourceDirection>+X</SourceDirection><FeatureName></FeatureName></SecondaryAxis></Value></Frame></Frames>  GraphicType=FromGeometry  MarkerShape=Sphere  MarkerSize=10  GraphicVisPropType=SimpleVisualProperties  GraphicDiffuseColor=[0.5 0.5 0.5]  GraphicSpecularColor=[0.5 0.5 0.5 1.0]  GraphicAmbientColor=[0.15 0.15 0.15 1.0]  GraphicEmissiveColor=[0.0 0.0 0.0 1.0]  GraphicShininess=75  GraphicOpacity=1.0
  Rigid Transform1 : sm_lib/Frames and Transforms/Rigid Transform  TranslationMethod=None  TranslationStandardOffset=22  TranslationStandardOffsetUnits=mm  TranslationStandardAxis=+Y  TranslationCartesianOffset=[0 0 0.22]  TranslationCartesianOffsetUnits=m  TranslationROffset=0  TranslationROffsetUnits=m  TranslationZOffset=0  TranslationZOffsetUnits=m  TranslationThetaOffset=0  TranslationThetaOffsetUnits=deg  RotationMethod=StandardAxis  RotationAngleUnits=deg  RotationStandardAxis=-X  RotationAngle=180  RotationArbitraryAxis=[0 0 1]  FollAlignAxisA=+X  BaseAlignAxisA=+Y  FollAlignAxisB=+Y  BaseAlignAxisB=+Z  RotationSequenceAxes=FollowerAxes  RotationSequence=XYX  RotationSequenceAngles=[0 0 0]  RotationSequenceAnglesUnits=deg  RotationMatrix=[1 0 0; 0 1 0; 0 0 1]  Quaternion=[1 0 0 0]
  Rigid Transform2 : sm_lib/Frames and Transforms/Rigid Transform  TranslationMethod=StandardAxis  TranslationStandardOffset=22  TranslationStandardOffsetUnits=mm  TranslationStandardAxis=-Z  TranslationCartesianOffset=[0 0 0.22]  TranslationCartesianOffsetUnits=m  TranslationROffset=0  TranslationROffsetUnits=m  TranslationZOffset=0  TranslationZOffsetUnits=m  TranslationThetaOffset=0  TranslationThetaOffsetUnits=deg  RotationMethod=None  RotationAngleUnits=deg  RotationStandardAxis=-Z  RotationAngle=180  RotationArbitraryAxis=[0 0 1]  FollAlignAxisA=+X  BaseAlignAxisA=+Y  FollAlignAxisB=+Y  BaseAlignAxisB=+Z  RotationSequenceAxes=FollowerAxes  RotationSequence=XYX  RotationSequenceAngles=[0 0 0]  RotationSequenceAnglesUnits=deg  RotationMatrix=[1 0 0; 0 1 0; 0 0 1]  Quaternion=[1 0 0 0]
  ThirdLinkJoint : sm_lib/Joints/Revolute Joint  JointMode=Normal  SenseConstraintForce=off  SenseConstraintForceX=off  SenseConstraintForceY=off  SenseConstraintForceZ=off  SenseConstraintTorque=off  SenseConstraintTorqueX=off  SenseConstraintTorqueY=off  SenseConstraintTorqueZ=off  SenseTotalForce=off  SenseTotalForceX=off  SenseTotalForceY=off  SenseTotalForceZ=off  SenseTotalTorque=off  SenseTotalTorqueX=off  SenseTotalTorqueY=off  SenseTotalTorqueZ=off  CompositeWrenchDir=FollowerOnBase  CompositeWrenchFrame=BaseFrame  EquilibriumPosition=0  EquilibriumPositionUnits=deg  SpringStiffness=0  SpringStiffnessUnits=N*m/deg  DampingCoefficient=0.1  DampingCoefficientUnits=N*m/(deg/s)  TorqueActuationMode=InputTorque  MotionActuationMode=ComputedMotion  SensePosition=on  SenseVelocity=on  SenseAcceleration=on  SenseTorqueForce=off  SenseLowerLimitTorqueForce=off  SenseUpperLimitTorqueForce=off  LowerLimitSpecify=on  LowerLimitBound=-110  LowerLimitBoundUnits=deg  LowerLimitStiffness=1e4  LowerLimitStiffnessUnits=N*m/deg  LowerLimitDamping=1000  LowerLimitDampingUnits=N*m/(deg/s)  LowerLimitTransitionRegionWidth=0.1  LowerLimitTransitionRegionWidthUnits=deg  UpperLimitSpecify=on  UpperLimitBound=155  UpperLimitBoundUnits=deg  UpperLimitStiffness=1e4  UpperLimitStiffnessUnits=N*m/deg  UpperLimitDamping=10  UpperLimitDampingUnits=N*m/(deg/s)  UpperLimitTransitionRegionWidth=0.1  UpperLimitTransitionRegionWidthUnits=deg  PositionTargetSpecify=on  PositionTargetPriority=High  PositionTargetValue=0  PositionTargetValueUnits=deg  VelocityTargetSpecify=off  VelocityTargetPriority=High  VelocityTargetValue=0  VelocityTargetValueUnits=deg/s
  Torque : PMIOPort  Side=Left
  PreviousLink : PMIOPort  Port=2  Side=Left
  Angle : PMIOPort  Port=3  Side=Right
  Velocity : PMIOPort  Port=4  Side=Right
  Acceleration : PMIOPort  Port=5  Side=Right
  NextLink : PMIOPort  Port=6  Side=Right
  connections:
  ThirdLinkJoint/RConn2 -- Angle/RConn1
  ThirdLinkJoint/RConn4 -- Acceleration/RConn1
  ThirdLinkJoint/RConn3 -- Velocity/RConn1
  NextLink/RConn1 -- FourthLinkBody/LConn1 -- ThirdLinkJoint/RConn1
  Rigid Transform2/RConn1 -- Rigid Transform1/LConn1
  Torque/RConn1 -- ThirdLinkJoint/LConn2
  Rigid Transform2/LConn1 -- PreviousLink/RConn1
  Rigid Transform1/RConn1 -- ThirdLinkJoint/LConn1

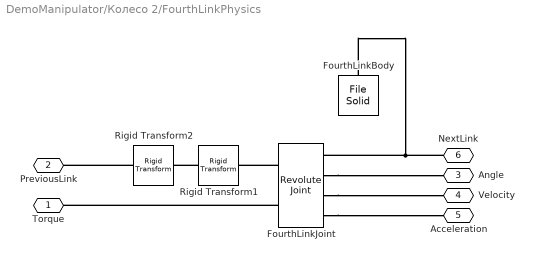
== system DemoManipulator/Колесо 2/FourthLinkPhysics ==
  FourthLinkBody : sm_lib/Body Elements/File Solid  ExtGeomFileName=C:\Users\Artem Sannikov\Desktop\Robo-Forester\Simulink_часть\3D_Models\Wheel.stp  UnitType=FromFile  ExtGeomFileUnits=m  StepReaderType=HEX  ExportConvexHullGeometry=off  InertiaType=Custom  Mass=1  MassUnits=kg  CenterOfMass=[0 0 -50]  CenterOfMassUnits=m  MomentsOfInertia=[5.7 15.3 4.1]  MomentsOfInertiaUnits=kg*m^2  ProductsOfInertia=[0 0 0]  ProductsOfInertiaUnits=kg*m^2  BasedOnType=DensityFromFile  Density=1000  DensityUnits=kg/m^3  DoExposeReferenceFrame=on  SerializedFrames=<Frames><Frame><Id>Frame1</Id><Value><Name>F1</Name><Origin><Source>GeometricFeature</Source><FeatureName>circular curve 3499</FeatureName></Origin><PrimaryAxis><DefinedDirection>+Z</DefinedDirection><Source>GeometricFeature</Source><SourceDirection>+Z</SourceDirection><FeatureName>segment 2464</FeatureName></PrimaryAxis><SecondaryAxis><DefinedDirection>+X</DefinedDirection><Source>ReferenceFrame</Source><SourceDirection>+X</SourceDirection><FeatureName></FeatureName></SecondaryAxis></Value></Frame></Frames>  GraphicType=FromGeometry  MarkerShape=Sphere  MarkerSize=10  GraphicVisPropType=SimpleVisualProperties  GraphicDiffuseColor=[0.5 0.5 0.5]  GraphicSpecularColor=[0.5 0.5 0.5 1.0]  GraphicAmbientColor=[0.15 0.15 0.15 1.0]  GraphicEmissiveColor=[0.0 0.0 0.0 1.0]  GraphicShininess=75  GraphicOpacity=1.0
  FourthLinkJoint : sm_lib/Joints/Revolute Joint  JointMode=Normal  SenseConstraintForce=off  SenseConstraintForceX=off  SenseConstraintForceY=off  SenseConstraintForceZ=off  SenseConstraintTorque=off  SenseConstraintTorqueX=off  SenseConstraintTorqueY=off  SenseConstraintTorqueZ=off  SenseTotalForce=off  SenseTotalForceX=off  SenseTotalForceY=off  SenseTotalForceZ=off  SenseTotalTorque=off  SenseTotalTorqueX=off  SenseTotalTorqueY=off  SenseTotalTorqueZ=off  CompositeWrenchDir=FollowerOnBase  CompositeWrenchFrame=BaseFrame  EquilibriumPosition=0  EquilibriumPositionUnits=deg  SpringStiffness=0  SpringStiffnessUnits=N*m/deg  DampingCoefficient=0.1  DampingCoefficientUnits=N*m/(deg/s)  TorqueActuationMode=InputTorque  MotionActuationMode=ComputedMotion  SensePosition=on  SenseVelocity=on  SenseAcceleration=on  SenseTorqueForce=off  SenseLowerLimitTorqueForce=off  SenseUpperLimitTorqueForce=off  LowerLimitSpecify=on  LowerLimitBound=-175  LowerLimitBoundUnits=deg  LowerLimitStiffness=1e4  LowerLimitStiffnessUnits=N*m/deg  LowerLimitDamping=1000  LowerLimitDampingUnits=N*m/(deg/s)  LowerLimitTransitionRegionWidth=0.1  LowerLimitTransitionRegionWidthUnits=deg  UpperLimitSpecify=on  UpperLimitBound=175  UpperLimitBoundUnits=deg  UpperLimitStiffness=1e4  UpperLimitStiffnessUnits=N*m/deg  UpperLimitDamping=10  UpperLimitDampingUnits=N*m/(deg/s)  UpperLimitTransitionRegionWidth=0.1  UpperLimitTransitionRegionWidthUnits=deg  PositionTargetSpecify=on  PositionTargetPriority=High  PositionTargetValue=0  PositionTargetValueUnits=deg  VelocityTargetSpecify=off  VelocityTargetPriority=High  VelocityTargetValue=0  VelocityTargetValueUnits=deg/s
  Rigid Transform1 : sm_lib/Frames and Transforms/Rigid Transform  TranslationMethod=None  TranslationStandardOffset=22  TranslationStandardOffsetUnits=mm  TranslationStandardAxis=+Y  TranslationCartesianOffset=[0 0 0.22]  TranslationCartesianOffsetUnits=m  TranslationROffset=0  TranslationROffsetUnits=m  TranslationZOffset=0  TranslationZOffsetUnits=m  TranslationThetaOffset=0  TranslationThetaOffsetUnits=deg  RotationMethod=StandardAxis  RotationAngleUnits=deg  RotationStandardAxis=-X  RotationAngle=180  RotationArbitraryAxis=[0 0 1]  FollAlignAxisA=+X  BaseAlignAxisA=+Y  FollAlignAxisB=+Y  BaseAlignAxisB=+Z  RotationSequenceAxes=FollowerAxes  RotationSequence=XYX  RotationSequenceAngles=[0 0 0]  RotationSequenceAnglesUnits=deg  RotationMatrix=[1 0 0; 0 1 0; 0 0 1]  Quaternion=[1 0 0 0]
  Rigid Transform2 : sm_lib/Frames and Transforms/Rigid Transform  TranslationMethod=StandardAxis  TranslationStandardOffset=22  TranslationStandardOffsetUnits=mm  TranslationStandardAxis=-Z  TranslationCartesianOffset=[0 0 0.22]  TranslationCartesianOffsetUnits=m  TranslationROffset=0  TranslationROffsetUnits=m  TranslationZOffset=0  TranslationZOffsetUnits=m  TranslationThetaOffset=0  TranslationThetaOffsetUnits=deg  RotationMethod=None  RotationAngleUnits=deg  RotationStandardAxis=-Z  RotationAngle=180  RotationArbitraryAxis=[0 0 1]  FollAlignAxisA=+X  BaseAlignAxisA=+Y  FollAlignAxisB=+Y  BaseAlignAxisB=+Z  RotationSequenceAxes=FollowerAxes  RotationSequence=XYX  RotationSequenceAngles=[0 0 0]  RotationSequenceAnglesUnits=deg  RotationMatrix=[1 0 0; 0 1 0; 0 0 1]  Quaternion=[1 0 0 0]
  Torque : PMIOPort  Side=Left
  PreviousLink : PMIOPort  Port=2  Side=Left
  Angle : PMIOPort  Port=3  Side=Right
  Velocity : PMIOPort  Port=4  Side=Right
  Acceleration : PMIOPort  Port=5  Side=Right
  NextLink : PMIOPort  Port=6  Side=Right
  connections:
  FourthLinkJoint/RConn2 -- Angle/RConn1
  FourthLinkJoint/RConn4 -- Acceleration/RConn1
  FourthLinkJoint/RConn3 -- Velocity/RConn1
  NextLink/RConn1 -- FourthLinkBody/LConn1 -- FourthLinkJoint/RConn1
  FourthLinkJoint/LConn2 -- Torque/RConn1
  FourthLinkJoint/LConn1 -- Rigid Transform1/RConn1
  Rigid Transform1/LConn1 -- Rigid Transform2/RConn1
  Rigid Transform2/LConn1 -- PreviousLink/RConn1
